simulink model "A1_cc"  (R2024a)
settings: Solver=ode45  StartTime=0.0  StopTime=100  MaxStep=1e-3  RelTol=1e-3
values from neighbouring files (symbols this model uses):
  a = data(2)    [A1_14.m]
  b = data(3)    [A1_14.m]
  g = 9.82    [A1_14.m]
  Ki = (2.25*m)/b    [A1_14.m]
  Kp = (m-a)/b    [A1_14.m]
  m = data(1)    [A1_14.m]
settings Model: Creator=jofr  LastModifiedBy=testuser
settings SolverCC: AlgebraicLoopSolver=TrustRegion
settings DataIOCC: LimitDataPoints=on  SaveFormat=Array  SignalLoggingSaveFormat=ModelDataLogs  ReturnWorkspaceOutputs=off
settings OptimizationCC: BlockReduction=off  BooleanDataType=off  LifeSpan=inf
settings DebuggingCC: SaveWithParameterizedLinksMsg=none  UnderspecifiedInitializationDetection=Classic  MergeDetectMultiDrivingBlocksExec=none  SignalResolutionControl=TryResolveAllWithWarning  MultiTaskDSMMsg=warning  MultiTaskCondExecSysMsg=none  UnconnectedInputMsg=warning  UnconnectedOutputMsg=warning  UnconnectedLineMsg=warning  SFUnexpectedBacktrackingDiag=warning  SFNoUnconditionalDefaultTransitionDiag=warning  SFExecutionAtInitializationDiag=none  ArithmeticOperatorsInVariantConditions=warning
settings HardwareCC: ProdBitPerPointer=32  ProdBitPerSizeT=32  ProdBitPerPtrDiffT=32  ProdLargestAtomicFloat=None  ProdIntDivRoundTo=Undefined  ProdEndianess=Unspecified  ProdWordSize=32  ProdHWDeviceType=32-bit Generic  TargetUnknown=on
settings ModelReferenceCC: EnableRefExpFcnMdlSchedulingChecks=on  PropagateSignalLabelsOutOfModel=off
settings SFSimCC: SimUseLocalCustomCode=off  CustomCodeUndefinedFunction=UseInterfaceOnly
settings RTWCC: RTWUseLocalCustomCode=off  GPUComputeCapability=3.5  DLArmComputeVersion=19.05
settings CodeAppCC: StateflowObjectComments=on
settings GRTTargetCC: TargetLangStandard=C89/C90 (ANSI)
settings ConfigComp: CovMetricSettings=dw  CovSaveCumulativeToWorkspaceVar=on  CovSaveSingleToWorkspaceVar=on  CovExternalEMLEnable=off

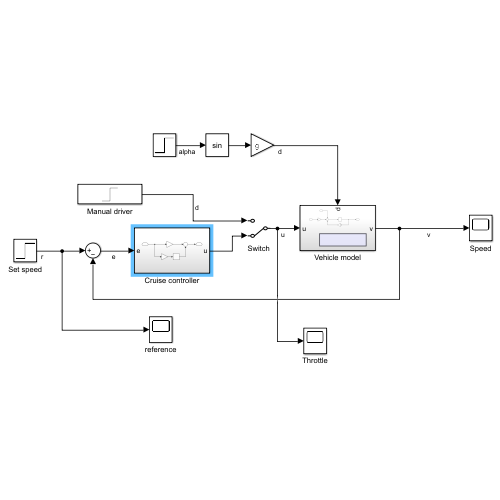
[thumbnail: Simulink's stored preview of the top-level diagram]
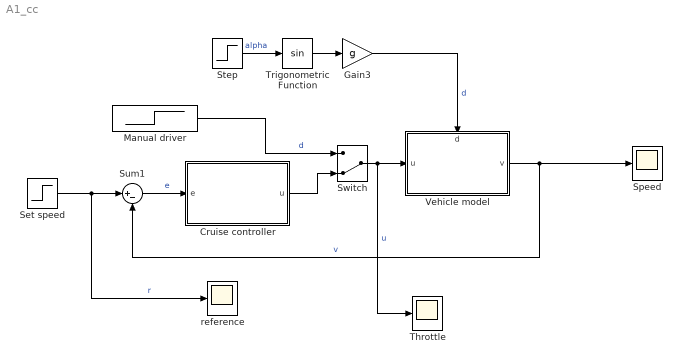
== system A1_cc ==
  Cruise controller : Subsystem
  Gain3 : Gain  Gain=g
  Manual driver : Step  Before=25*a/b  After=30*a/b  SampleTime=0
  Set speed : Step  Before=25  After=30  SampleTime=0
  Speed : Scope
  Step : Step  Time=1000  After=0.1  SampleTime=0
  Sum1 : Sum  Inputs=|+-
  Switch : ManualSwitch  CurrentSetting=0
  Throttle : Scope
  Trigonometric Function : Trigonometry
  Vehicle model : Subsystem
      settings: PortSchema="{\"entries\":[{\"content\":{\"sides\":[{\"content\":{\"connectorIds\":[\"In1\"]},\"type\":\"ConnectorPlacement.EquallySpacedRectSide\",\"uuid\":\"8188ec2e-7b14-4fd6-ab55-7cea6e9f54e2\"},{\"content\":{\"connectorIds\":[\"Out1\"],\"side\":\"RIGHT\"},\"type\":\"ConnectorPlacement.EquallySpacedRectSide\",\"uuid\":\"403e2e46-1697-4bb6-98fa-f8a08edec7c4\"},{\"content\":{\"connectorIds\":[\"In2\"],\"side\":\"TOP\"},\"type\":\"ConnectorPlacement.EquallySpacedRectSide\",\"uuid\":\"1cc5364f-c05a-4d3f-ac94-5b665fe415b4\"},{\"content\":{\"connectorIds\":[],\"side\":\"HIDDEN\"},\"type\":\"ConnectorPlacement.EquallySpacedRectSide\",\"uuid\":\"4fc64fe0-eaad-4a3e-850d-8e1dbe967cca\"}]},\"type\":\"ConnectorPlacement.EquallySpacedConnector\",\"uuid\":\"84be3d81-93f1-400b-9ab2-2fcef574c47e\"}],\"packageUris\":[\"http://schema.mathworks.com/mf0/Connector/R2020b\"],\"version\":\"1.0\"}"
  reference : Scope
  wires:
  Trigonometric Function/1 -> Gain3/1
  Step/1 -> Trigonometric Function/1  "alpha"
  Set speed/1 -> Sum1/1, reference/1  "r"
  Sum1/1 -> Cruise controller/1(e)  "e"
  Vehicle model/1(v) -> Sum1/2, Speed/1  "v"
  Gain3/1 -> Vehicle model/2(d)  "d"
  Switch/1 -> Throttle/1, Vehicle model/1(u)  "u"
  Cruise controller/1(u) -> Switch/2
  Manual driver/1 -> Switch/1  "d"

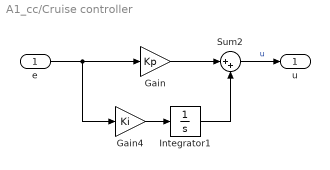
== system A1_cc/Cruise controller ==
  e : Inport
  Gain : Gain  Gain=Kp
  Gain4 : Gain  Gain=Ki
  Integrator1 : Integrator  InitialCondition=a*25/b
  Sum2 : Sum  Inputs=|++
  u : Outport
  wires:
  Gain4/1 -> Integrator1/1
  Gain/1 -> Sum2/1
  Sum2/1 -> u/1  "u"
  Integrator1/1 -> Sum2/2
  e/1 -> Gain4/1, Gain/1

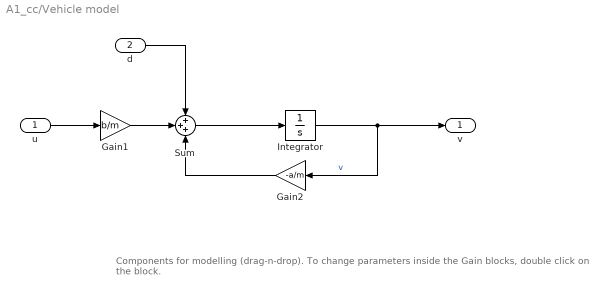
== system A1_cc/Vehicle model ==
  note: Components for modelling (drag-n-drop). To change parameters inside the
      | Gain blocks, double click on the block.
  u : Inport
  d : Inport  Port=2
  Gain1 : Gain  Gain=b/m
  Gain2 : Gain  Gain=-a/m
  Integrator : Integrator  InitialCondition=25
  Sum : Sum  Inputs=+++
  v : Outport
  wires:
  u/1 -> Gain1/1
  Gain1/1 -> Sum/2
  Sum/1 -> Integrator/1
  Integrator/1 -> Gain2/1, v/1  "v"
  Gain2/1 -> Sum/3
  d/1 -> Sum/1
